simulink model "serial3_multibody_dynamixel"  (R2021a)
settings: Solver=VariableStepAuto  StartTime=0.0  StopTime=10  RelTol=1e-3
undefined symbols (not defined in the file or in its folder): smiData, X, Y, Z
libraries: sm_lib x134, slDxl_lib x14, simulink_extras x6, nesl_utility x4
(part 3 of 3)

== system serial3_multibody_dynamixel/Representacion en Multibody/E3_3_1_RIGID/EnsamblajeTubo15_1_RIGID/BaseTubo_1_RIGID ==
  ReferenceFrame : sm_lib/Frames and Transforms/Reference Frame
  Solid : sm_lib/Body Elements/File Solid  ExtGeomFileName=BaseTubo_Predeterminado_sldprt.STEP  UnitType=FromFile  ExtGeomFileUnits=m  StepReaderType=HEX  ExportConvexHullGeometry=off  InertiaType=Custom  Mass=smiData.Solid(7).mass  MassUnits=kg  CenterOfMass=smiData.Solid(7).CoM  CenterOfMassUnits=cm  MomentsOfInertia=smiData.Solid(7).MoI  MomentsOfInertiaUnits=kg*cm^2  ProductsOfInertia=smiData.Solid(7).PoI  ProductsOfInertiaUnits=kg*cm^2  BasedOnType=Density  Density=1000  DensityUnits=kg/m^3  DoExposeReferenceFrame=on  SerializedFrames=<Frames/>  GraphicType=FromGeometry  MarkerShape=Sphere  MarkerSize=10  GraphicVisPropType=SimpleVisualProperties  GraphicDiffuseColor=smiData.Solid(7).color  GraphicSpecularColor=[0.5 0.5 0.5 1.0]  GraphicAmbientColor=[0.15 0.15 0.15 1.0]  GraphicEmissiveColor=[0.0 0.0 0.0 1.0]  GraphicShininess=75  GraphicOpacity=smiData.Solid(7).opacity
  F : PMIOPort  Side=Left
  connections:
  Solid/RConn1 -- ReferenceFrame/RConn1 -- F/RConn1

== system serial3_multibody_dynamixel/Representacion en Multibody/E3_3_1_RIGID/EnsamblajeTubo15_1_RIGID/BaseTubo_2_RIGID ==
  ReferenceFrame : sm_lib/Frames and Transforms/Reference Frame
  Solid : sm_lib/Body Elements/File Solid  ExtGeomFileName=BaseTubo_Predeterminado_sldprt.STEP  UnitType=FromFile  ExtGeomFileUnits=m  StepReaderType=HEX  ExportConvexHullGeometry=off  InertiaType=Custom  Mass=smiData.Solid(7).mass  MassUnits=kg  CenterOfMass=smiData.Solid(7).CoM  CenterOfMassUnits=cm  MomentsOfInertia=smiData.Solid(7).MoI  MomentsOfInertiaUnits=kg*cm^2  ProductsOfInertia=smiData.Solid(7).PoI  ProductsOfInertiaUnits=kg*cm^2  BasedOnType=Density  Density=1000  DensityUnits=kg/m^3  DoExposeReferenceFrame=on  SerializedFrames=<Frames/>  GraphicType=FromGeometry  MarkerShape=Sphere  MarkerSize=10  GraphicVisPropType=SimpleVisualProperties  GraphicDiffuseColor=smiData.Solid(7).color  GraphicSpecularColor=[0.5 0.5 0.5 1.0]  GraphicAmbientColor=[0.15 0.15 0.15 1.0]  GraphicEmissiveColor=[0.0 0.0 0.0 1.0]  GraphicShininess=75  GraphicOpacity=smiData.Solid(7).opacity
  F : PMIOPort  Side=Left
  connections:
  Solid/RConn1 -- ReferenceFrame/RConn1 -- F/RConn1

== system serial3_multibody_dynamixel/Representacion en Multibody/E3_3_1_RIGID/EnsamblajeTubo15_1_RIGID/Tubo15cm_1_RIGID ==
  ReferenceFrame : sm_lib/Frames and Transforms/Reference Frame
  Solid : sm_lib/Body Elements/File Solid  ExtGeomFileName=Tubo15cm_Predeterminado_sldprt.STEP  UnitType=FromFile  ExtGeomFileUnits=m  StepReaderType=HEX  ExportConvexHullGeometry=off  InertiaType=Custom  Mass=smiData.Solid(6).mass  MassUnits=kg  CenterOfMass=smiData.Solid(6).CoM  CenterOfMassUnits=cm  MomentsOfInertia=smiData.Solid(6).MoI  MomentsOfInertiaUnits=kg*cm^2  ProductsOfInertia=smiData.Solid(6).PoI  ProductsOfInertiaUnits=kg*cm^2  BasedOnType=Density  Density=1000  DensityUnits=kg/m^3  DoExposeReferenceFrame=on  SerializedFrames=<Frames/>  GraphicType=FromGeometry  MarkerShape=Sphere  MarkerSize=10  GraphicVisPropType=SimpleVisualProperties  GraphicDiffuseColor=smiData.Solid(6).color  GraphicSpecularColor=[0.5 0.5 0.5 1.0]  GraphicAmbientColor=[0.15 0.15 0.15 1.0]  GraphicEmissiveColor=[0.0 0.0 0.0 1.0]  GraphicShininess=75  GraphicOpacity=smiData.Solid(6).opacity
  F : PMIOPort  Side=Left
  connections:
  Solid/RConn1 -- ReferenceFrame/RConn1 -- F/RConn1

== matlab function serial3_multibody_dynamixel/Dinamica Directa ==
  data: q1 input; q1pp output; q2 input; q3 input; q1p input; q2p input; q3p input; tau1 input; tau2 input; tau3 input; q2pp output; q3pp output
function [q1pp,q2pp,q3pp] = din_directa(q1,q2,q3,q1p,q2p,q3p,tau1,tau2,tau3)

M =[ (5589*cos(q3))/20000000 - (833252400176387296733*cos(2*q2))/5764607523034234880000000 - (12569150243223845732103*cos(2*q2 + 2*q3))/92233720368547758080000000 - (5589*cos(2*q2 + q3))/20000000 + 51717330115768924042331/92233720368547758080000000,                                    0,                                     0;
                                                                                                                                                                                                                                                   0, 5676674199877871/4611686018427387904,  5351169871482219/9223372036854775808;
                                                                                                                                                                                                                                                 0, 5351169871482219/9223372036854775808, 5547397111566305/18446744073709551616];
 
G =[0;-(42678181724791417*sin(q2+q3))/1801439850948198400-(3884277835938411*sin(q2))/28147497671065600;-(6828509075966627*sin(q2 + q3))/288230376151711744];
 
 
C = [q1p*((833252400176387296733*q2p*sin(2*q2))/2882303761517117440000000 + (12569150243223845732103*q2p*sin(2*q2 + 2*q3))/46116860184273879040000000 + (12569150243223845732103*q3p*sin(2*q2 + 2*q3))/46116860184273879040000000 - (5589*q3p*sin(q3))/20000000 + (5589*q2p*sin(2*q2 + q3))/10000000 + (5589*q3p*sin(2*q2 + q3))/20000000);
                                                                                                                                                     -(q1p^2*((5589*sin(2*q2 + q3))/10000000 + (833252400176387296733*sin(2*q2))/2882303761517117440000000 + (12569150243223845732103*sin(2*q2 + 2*q3))/46116860184273879040000000))/2;
                                                                                                                                                                                         -(q1p^2*((5589*sin(2*q2 + q3))/20000000 + (12569150243223845732103*sin(2*q2 + 2*q3))/46116860184273879040000000 - (5589*sin(q3))/20000000))/2];
Fm1=0.123;
F=[Fm1*q1p;Fm1*q2p;Fm1*q3p];    %Friccion de las juntas - Funcion disipativa

Tau=[tau1;tau2;tau3];
qpp=(inv(M))*(Tau-C-G-F);
q1pp=qpp(1);
q2pp=qpp(2);
q3pp=qpp(3);

== matlab function serial3_multibody_dynamixel/Control PD ==
  data: q1 input; tau1 output; q2 input; q3 input; q1d input; q2d input; q3d input; q1p input; q2p input; q3p input; tau2 output; tau3 output
function [tau1,tau2,tau3] = controlpd(q1,q2,q3,q1d,q2d,q3d,q1p,q2p,q3p)

kp=1;
kv=0.02;

Kp=[kp 0 0;0 kp 0;0 0 kp];
Kv=[kv 0 0;0 kv 0;0 0 kv];

qe=[q1d-q1;q2d-q2;q3d-q3];

qp=[q1;q2;q3];

G =[0;-(42678181724791417*sin(q2+q3))/1801439850948198400-(3884277835938411*sin(q2))/28147497671065600;-(6828509075966627*sin(q2 + q3))/288230376151711744];
 
Tau=Kp*qe-Kv*qp+G;
tau1=Tau(1);
tau2=Tau(2);
tau3=Tau(3);
